simulink model "grid"  (R2023b)
settings: Solver=VariableStepAuto  StartTime=0.1  StopTime=180  RelTol=1e-3
values from neighbouring files (symbols this model uses):
  close_time = 40    [params.m]
  M1 = M1_backup    [automation.m]    (also in params.m = Machine)
  M2 = M1    [automation.m]    (also in params.m = Machine)
  open_time = 80    [params.m]
  Pn_L1 = M1.P0 + M2.P0    [params.m]
  Pn_L2 = Pn_L1 * 0.2    [params.m]
libraries: nesl_utility x21, ee_lib x21, fl_lib x10
settings Model: Creator=gosmann  LastModifiedBy=felipe

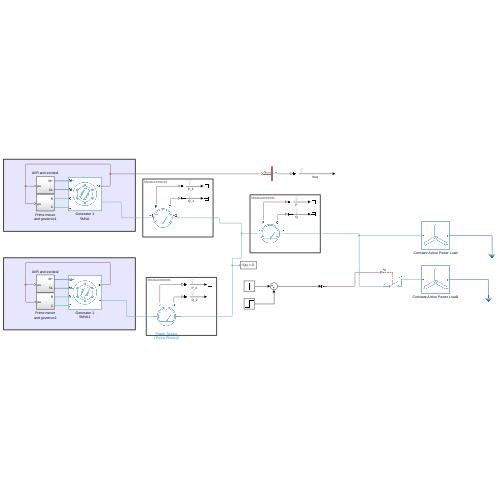
[thumbnail: Simulink's stored preview of the top-level diagram]
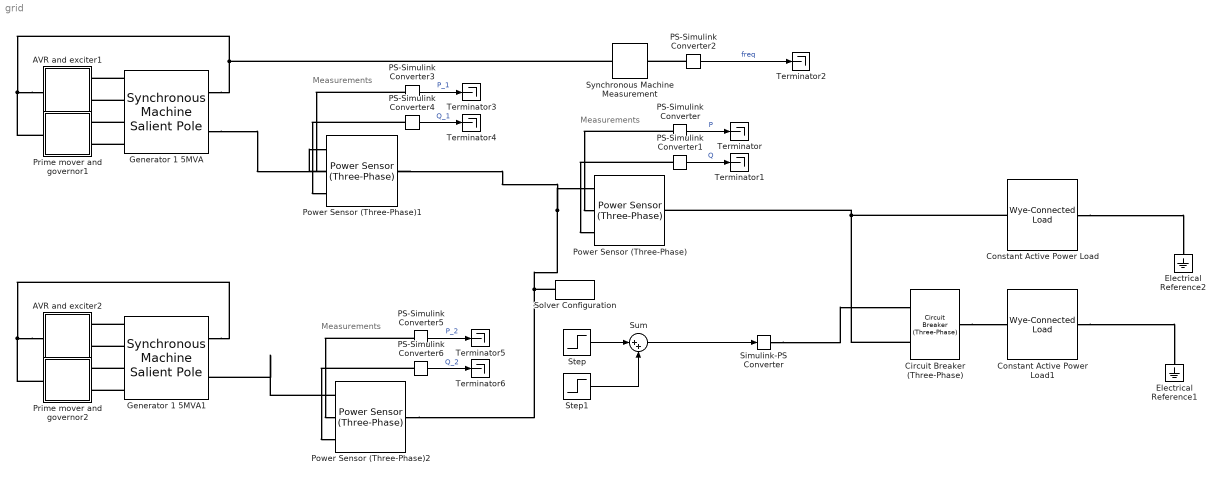
== system grid ==
  note: Measurements
  note: Measurements
  note: Measurements
  AVR and exciter1 : Subsystem
  AVR and exciter2 : Subsystem
  Circuit Breaker (Three-Phase) : ee_lib/Switches & Breakers/Circuit Breaker (Three-Phase)  R_closed=0.001 Ohm  G_open=1e-6 1/Ohm  threshold=0.5 V  breaker_behavior=ee.enum.switches.breakerBehavior.zeroCrossingEnable
      settings: InternalSimscapePortConfiguration="{\"Bottom\":[],\"Left\":[{\"id\":\"vT\",\"label\":\"vT\",\"type\":\"input\"},{\"id\":\"N1\",\"label\":\"~1\",\"type\":\"foundation.electrical.three_phase\"}],\"Right\":[{\"id\":\"N2\",\"label\":\"~2\",\"type\":\"foundation.electrical.three_phase\"}],\"Top\":[]}"
  Constant Active Power Load : ee_lib/Passive/RLC Assemblies/Wye-Connected Load  parameterization=ee.enum.rlc.parameterization.ratedpower  component_structure=ee.enum.rlc.structure.L  component_structure_PQ=ee.enum.rlc.structure.R  R=1 Ohm  L=7.3478 H  C=1e-6 F  VRated=ref_volt V  FRated=60 Hz  P=Pn_L1 W  Qpos=6000 A*V  Qneg=-1e2 A*V  R_parasitic=0 Ohm  G_parasitic=0 1/Ohm  R_parasitic_PQ=0 Ohm  G_parasitic_PQ=0 1/Ohm  Vmag0=4160*0.98 V  Vang0=0 deg  Freq0=60 Hz  IL_specify=off  IL_priority=High  IL=[0, 0, 0] A  IL_nominal_specify=off  IL_nominal_unit=A  IL_nominal_value=1  VC_specify=off  VC_priority=High  VC=[0, 0, 0] V  VC_nominal_specify=off  VC_nominal_unit=V  VC_nominal_value=1
  Constant Active Power Load1 : ee_lib/Passive/RLC Assemblies/Wye-Connected Load  parameterization=ee.enum.rlc.parameterization.ratedpower  component_structure=ee.enum.rlc.structure.L  component_structure_PQ=ee.enum.rlc.structure.R  R=1 Ohm  L=7.3478 H  C=1e-6 F  VRated=ref_volt V  FRated=60 Hz  P=Pn_L2 W  Qpos=6000 A*V  Qneg=-1e2 A*V  R_parasitic=0 Ohm  G_parasitic=0 1/Ohm  R_parasitic_PQ=0 Ohm  G_parasitic_PQ=0 1/Ohm  Vmag0=4160*0.98 V  Vang0=0 deg  Freq0=60 Hz  IL_specify=off  IL_priority=High  IL=[0, 0, 0] A  IL_nominal_specify=off  IL_nominal_unit=A  IL_nominal_value=1  VC_specify=off  VC_priority=High  VC=[0, 0, 0] V  VC_nominal_specify=off  VC_nominal_unit=V  VC_nominal_value=1
  Electrical Reference1 : fl_lib/Electrical/Electrical Elements/Electrical Reference
  Electrical Reference2 : fl_lib/Electrical/Electrical Elements/Electrical Reference
  Generator 1 5MVA : ee_lib/Electromechanical/Synchronous/Synchronous Machine Salient Pole  port_option=ee.enum.threePhasePort.composite  SRated=M1.Pn A*V  VRated=ref_volt V  FRated=ref_freq Hz  nPolePairs=M1.pole_pairs  param_option=ee.enum.sm.parameterization.standard  fieldCircuitParameterization_option=ee.enum.sm.fieldparameterization.current  baseEfd=216.54 V  baseIfd=M1.field_In A  zero_sequence=ee.enum.park.zerosequence.exclude  axes_param=ee.enum.rotorangle.daxis  Ladu=0.9  Laqu=0.55  L0=0.15  Ll=0.15  Ra=M1.Ra  Lfd=0.2571  Rfd=0.0006  L1d=0.2  R1d=0.0354  L1q=0.2567  R1q=0.0428  Xl=M1.Xi  Xd=M1.Xd  Xq=M1.Xq  X0=0.15  Xdd=M1.Xd_l  Xddd=M1.Xd_ll  Xqdd=M1.Xq_ll  d_option=ee.enum.circuit.open  Td0d=M1.Td0_l s  Tdd=1.75 s  Td0dd=M1.Td0_ll s  Tddd=0.0214 s  q_option=ee.enum.circuit.open  Tq0dd=M1.Tq0_ll s  Tqdd=0.0232 s  saturation_option=ee.enum.saturation.exclude  saturation_ifd=[0.00, 0.48, 0.76, 1.38, 1.79]  saturation_Vag=[0.00, 0.43, 0.59, 0.71, 0.76]  initialization_option=ee.enum.sm.initialization.electrical  source_type=ee.enum.sm.load_flow_source_type.Swing  Vmag0=ref_volt V  Vang0=0 deg  Pt0=M1.P0 A*V  Qt0=0 A*V  minimum_pu=0.95  phase_search_range=[-inf, inf] deg  gmin=1e-6 S  connection_option=ee.enum.Connection.wye  num_q_dampers=1  rotor_offset=-pi / 2 rad  pu_psid_specify=on  pu_psid_priority=High  pu_psid=0  pu_psid_nominal_specify=off  pu_psid_nominal_unit=1  pu_psid_nominal_value=1  pu_psiq_specify=on  pu_psiq_priority=High  pu_psiq=0  pu_psiq_nominal_specify=off  pu_psiq_nominal_unit=1  pu_psiq_nominal_value=1  pu_psifd_specify=on  pu_psifd_priority=High  pu_psifd=0  pu_psifd_nominal_specify=off  pu_psifd_nominal_unit=1  pu_psifd_nominal_value=1  pu_psi1d_specify=on  pu_psi1d_priority=High  pu_psi1d=0  pu_psi1d_nominal_specify=off  pu_psi1d_nominal_unit=1  pu_psi1d_nominal_value=1  pu_psi1q_specify=on  pu_psi1q_priority=High  pu_psi1q=0  pu_psi1q_nominal_specify=off  pu_psi1q_nominal_unit=1  pu_psi1q_nominal_value=1  angular_position_diff_specify=on  angular_position_diff_priority=High  angular_position_diff=0 deg  angular_position_diff_nominal_specify=off  angular_position_diff_nominal_unit=deg  angular_position_diff_nominal_value=1  Tmeas=298.15 K  alpha=3.93e-3 1/K  stator_thermal_mass=100 J/K  rotor_thermal_mass=200 J/K  temperatureA_specify=off  temperatureA_priority=High  temperatureA=25 degC  temperatureA_nominal_specify=off  temperatureA_nominal_unit=degC  temperatureA_nominal_value=1  temperatureB_specify=off  temperatureB_priority=High  temperatureB=25 degC  temperatureB_nominal_specify=off  temperatureB_nominal_unit=degC  temperatureB_nominal_value=1  temperatureC_specify=off  temperatureC_priority=High  temperatureC=25 degC  temperatureC_nominal_specify=off  temperatureC_nominal_unit=degC  temperatureC_nominal_value=1  temperatureR_specify=off  temperatureR_priority=High  temperatureR=25 degC  temperatureR_nominal_specify=off  temperatureR_nominal_unit=degC  temperatureR_nominal_value=1
      settings: LogSimulationData=on  InternalSimscapePortConfiguration="{\"Bottom\":[],\"Left\":[{\"id\":\"fd_p\",\"label\":\"fd+\",\"type\":\"foundation.electrical.electrical\"},{\"id\":\"fd_n\",\"label\":\"fd-\",\"type\":\"foundation.electrical.electrical\"},{\"id\":\"R\",\"label\":\"R\",\"type\":\"foundation.mechanical.rotational.rotational\"},{\"id\":\"C\",\"label\":\"C\",\"type\":\"foundation.mechanical.rotational.rotational\"}],\"Right\":[{\"id\":\"pu_output\",\"label\":\"pu\",\"type\":\"output\"},{\"id\":\"N\",\"label\":\"~\",\"type\":\"foundation.electrical.three_phase\"}],\"Top\":[]}"
  Generator 1 5MVA1 : ee_lib/Electromechanical/Synchronous/Synchronous Machine Salient Pole  port_option=ee.enum.threePhasePort.composite  SRated=M2.Pn A*V  VRated=ref_volt V  FRated=ref_freq Hz  nPolePairs=M2.pole_pairs  param_option=ee.enum.sm.parameterization.standard  fieldCircuitParameterization_option=ee.enum.sm.fieldparameterization.current  baseEfd=216.54 V  baseIfd=M2.field_In A  zero_sequence=ee.enum.park.zerosequence.exclude  axes_param=ee.enum.rotorangle.daxis  Ladu=0.9  Laqu=0.55  L0=0.15  Ll=0.15  Ra=M2.Ra  Lfd=0.2571  Rfd=0.0006  L1d=0.2  R1d=0.0354  L1q=0.2567  R1q=0.0428  Xl=M2.Xi  Xd=M2.Xd  Xq=M2.Xq  X0=0.15  Xdd=M2.Xd_l  Xddd=M2.Xd_ll  Xqdd=M2.Xq_ll  d_option=ee.enum.circuit.open  Td0d=M2.Td0_l s  Tdd=1.75 s  Td0dd=M2.Td0_ll s  Tddd=0.0214 s  q_option=ee.enum.circuit.open  Tq0dd=M2.Tq0_ll s  Tqdd=0.0232 s  saturation_option=ee.enum.saturation.exclude  saturation_ifd=[0.00, 0.48, 0.76, 1.38, 1.79]  saturation_Vag=[0.00, 0.43, 0.59, 0.71, 0.76]  initialization_option=ee.enum.sm.initialization.electrical  source_type=ee.enum.sm.load_flow_source_type.Swing  Vmag0=ref_volt V  Vang0=0 deg  Pt0=M2.P0 A*V  Qt0=0 A*V  minimum_pu=0.95  phase_search_range=[-inf, inf] deg  gmin=1e-6 S  connection_option=ee.enum.Connection.wye  num_q_dampers=1  rotor_offset=-pi / 2 rad  pu_psid_specify=on  pu_psid_priority=High  pu_psid=0  pu_psid_nominal_specify=off  pu_psid_nominal_unit=1  pu_psid_nominal_value=1  pu_psiq_specify=on  pu_psiq_priority=High  pu_psiq=0  pu_psiq_nominal_specify=off  pu_psiq_nominal_unit=1  pu_psiq_nominal_value=1  pu_psifd_specify=on  pu_psifd_priority=High  pu_psifd=0  pu_psifd_nominal_specify=off  pu_psifd_nominal_unit=1  pu_psifd_nominal_value=1  pu_psi1d_specify=on  pu_psi1d_priority=High  pu_psi1d=0  pu_psi1d_nominal_specify=off  pu_psi1d_nominal_unit=1  pu_psi1d_nominal_value=1  pu_psi1q_specify=on  pu_psi1q_priority=High  pu_psi1q=0  pu_psi1q_nominal_specify=off  pu_psi1q_nominal_unit=1  pu_psi1q_nominal_value=1  angular_position_diff_specify=on  angular_position_diff_priority=High  angular_position_diff=0 deg  angular_position_diff_nominal_specify=off  angular_position_diff_nominal_unit=deg  angular_position_diff_nominal_value=1  Tmeas=298.15 K  alpha=3.93e-3 1/K  stator_thermal_mass=100 J/K  rotor_thermal_mass=200 J/K  temperatureA_specify=off  temperatureA_priority=High  temperatureA=25 degC  temperatureA_nominal_specify=off  temperatureA_nominal_unit=degC  temperatureA_nominal_value=1  temperatureB_specify=off  temperatureB_priority=High  temperatureB=25 degC  temperatureB_nominal_specify=off  temperatureB_nominal_unit=degC  temperatureB_nominal_value=1  temperatureC_specify=off  temperatureC_priority=High  temperatureC=25 degC  temperatureC_nominal_specify=off  temperatureC_nominal_unit=degC  temperatureC_nominal_value=1  temperatureR_specify=off  temperatureR_priority=High  temperatureR=25 degC  temperatureR_nominal_specify=off  temperatureR_nominal_unit=degC  temperatureR_nominal_value=1
      settings: LogSimulationData=on  InternalSimscapePortConfiguration="{\"Bottom\":[],\"Left\":[{\"id\":\"fd_p\",\"label\":\"fd+\",\"type\":\"foundation.electrical.electrical\"},{\"id\":\"fd_n\",\"label\":\"fd-\",\"type\":\"foundation.electrical.electrical\"},{\"id\":\"R\",\"label\":\"R\",\"type\":\"foundation.mechanical.rotational.rotational\"},{\"id\":\"C\",\"label\":\"C\",\"type\":\"foundation.mechanical.rotational.rotational\"}],\"Right\":[{\"id\":\"pu_output\",\"label\":\"pu\",\"type\":\"output\"},{\"id\":\"N\",\"label\":\"~\",\"type\":\"foundation.electrical.three_phase\"}],\"Top\":[]}"
  PS-Simulink Converter{,1,3..6} (6 alike) : nesl_utility/PS-Simulink Converter  PhysicalDomain=network_engine_domain  SubClassName=ps_output  LeftPortType=input  RightPortType=output  PseudoPeriodic=off  Frequencies=[]  VectorFormat=1-D array  Unit=inherit  AffineConversion=off
  PS-Simulink Converter2 : nesl_utility/PS-Simulink Converter  PhysicalDomain=network_engine_domain  SubClassName=ps_output  LeftPortType=input  RightPortType=output  PseudoPeriodic=off  Frequencies=[]  VectorFormat=inherit  Unit=inherit  AffineConversion=off
  Power Sensor (Three-Phase) : ee_lib/Sensors & Transducers/Power Sensor (Three-Phase)  load_type=ee.enum.passive.type_balanced.balanced  f0=60 Hz  config=ee.enum.with_neutral.no  rho=1
      settings: InternalSimscapePortConfiguration="{\"Bottom\":[],\"Left\":[{\"id\":\"N1\",\"label\":\"~1\",\"type\":\"foundation.electrical.three_phase\"}],\"Right\":[{\"id\":\"N2\",\"label\":\"~2\",\"type\":\"foundation.electrical.three_phase\"}],\"Top\":[{\"id\":\"Pm\",\"label\":\"P\",\"type\":\"output\"},{\"id\":\"Qm\",\"label\":\"Q\",\"type\":\"output\"}]}"
  Power Sensor (Three-Phase)1 : ee_lib/Sensors & Transducers/Power Sensor (Three-Phase)  load_type=ee.enum.passive.type_balanced.balanced  f0=60 Hz  config=ee.enum.with_neutral.no  rho=1
      settings: InternalSimscapePortConfiguration="{\"Bottom\":[],\"Left\":[{\"id\":\"N1\",\"label\":\"~1\",\"type\":\"foundation.electrical.three_phase\"}],\"Right\":[{\"id\":\"N2\",\"label\":\"~2\",\"type\":\"foundation.electrical.three_phase\"}],\"Top\":[{\"id\":\"Pm\",\"label\":\"P\",\"type\":\"output\"},{\"id\":\"Qm\",\"label\":\"Q\",\"type\":\"output\"}]}"
  Power Sensor (Three-Phase)2 : ee_lib/Sensors & Transducers/Power Sensor (Three-Phase)  load_type=ee.enum.passive.type_balanced.balanced  f0=60 Hz  config=ee.enum.with_neutral.no  rho=1
      settings: InternalSimscapePortConfiguration="{\"Bottom\":[],\"Left\":[{\"id\":\"N1\",\"label\":\"~1\",\"type\":\"foundation.electrical.three_phase\"}],\"Right\":[{\"id\":\"N2\",\"label\":\"~2\",\"type\":\"foundation.electrical.three_phase\"}],\"Top\":[{\"id\":\"Pm\",\"label\":\"P\",\"type\":\"output\"},{\"id\":\"Qm\",\"label\":\"Q\",\"type\":\"output\"}]}"
  Prime mover and governor1 : Subsystem
  Prime mover and governor2 : Subsystem
  Simulink-PS Converter : nesl_utility/Simulink-PS Converter  PhysicalDomain=network_engine_domain  SubClassName=ps_input  LeftPortType=input  RightPortType=output  PseudoPeriodic=off  Frequencies=[]  NoiseDistribution=none  NoiseParameters=[]  Unit=1  AffineConversion=off  FilteringAndDerivatives=provide  SimscapeFilterOrder=1  InputFilterTimeConstant=0.001  UdotUserProvided=0
  Solver Configuration : nesl_utility/Solver Configuration  PhysicalDomain=network_engine_domain  SubClassName=solver  LeftPortType=input  RightPortType=generic  Tones=[]  Harmonics=[]  SimulateNoise=off  Profile=off  UseLocalSampling=off  EnableSwitchedLinearOptims=on  FrequencyDomain=off  UseCCode=off  RelTol=0.001  AbsTol=1e-06  MinStep=1e-09  ToWorkspace=off  RevertToSquareIcSolve=off  NumHomotopyIterations=100  PhasorMode=off  PhasorModeNumHarmonics=1  ConsistencySolver=NEWTON_FTOL  IndexReductionMethod=DerivativeReplacement  DoDC=off  ResidualTolerance=1e-09  ConsistencyTolSource=GLOBAL  ConsistencyAbsTol=0.001  ConsistencyRelTol=0.001  ConsistencyTolFactor=0.001  UseLocalSolver=on  LocalSolverChoice=NE_TRAPEZOIDAL_ADVANCER  ResolveIndetEquations=on  FunctionEvalNumThread=1  LocalSolverSampleTime=2e-4  DoFixedCost=on  MaxNonlinIter=1  MaxModeIter=2  ComputeImpulses=off  ImpulseIterations=1  LinearAlgebra=Full  LinearAlgebraNumThread=0  EquationFormulation=NE_TIME_EF  DelaysMemoryBudget=1024  AutomaticFiltering=on  FilteringTimeConstant=0.001  PartitionStorageMethod=AS_NEEDED  PartitionMemoryBudget=1024  PartitionMethod=ROBUST  MultibodyUseLocalSolver=off  MultibodyLocalSolverChoice=ODE1  MultibodyLocalSolverSampleTime=0.001
  Step : Step  Time=close_time  Before=1  After=0  SampleTime=0
  Step1 : Step  Time=open_time  SampleTime=0
  Sum : Sum  Inputs=|++
  Synchronous Machine Measurement : ee_lib/Electromechanical/Synchronous/Synchronous Machine Measurement  output_idx=4
      settings: InternalSimscapePortConfiguration="{\"Bottom\":[],\"Left\":[{\"id\":\"pu_input\",\"label\":\"pu\",\"type\":\"input\"}],\"Right\":[{\"id\":\"pu_output\",\"label\":\"o\",\"type\":\"output\"}],\"Top\":[]}"
  Terminator{,1..6} (7 alike) : Terminator
  wires:
  PS-Simulink Converter1/1 -> Terminator1/1  "Q"
  PS-Simulink Converter/1 -> Terminator/1  "P"
  PS-Simulink Converter2/1 -> Terminator2/1  "freq"
  Step/1 -> Sum/1
  Sum/1 -> Simulink-PS Converter/1
  Step1/1 -> Sum/2
  PS-Simulink Converter3/1 -> Terminator3/1  "P_1"
  PS-Simulink Converter4/1 -> Terminator4/1  "Q_1"
  PS-Simulink Converter5/1 -> Terminator5/1  "P_2"
  PS-Simulink Converter6/1 -> Terminator6/1  "Q_2"
  connections:
  Constant Active Power Load/LConn1 -- Circuit Breaker (Three-Phase)/LConn2 -- Power Sensor (Three-Phase)/RConn1
  Constant Active Power Load/RConn1 -- Electrical Reference2/LConn1
  PS-Simulink Converter/LConn1 -- Power Sensor (Three-Phase)/LConn2
  PS-Simulink Converter1/LConn1 -- Power Sensor (Three-Phase)/LConn3
  PS-Simulink Converter2/LConn1 -- Synchronous Machine Measurement/RConn1
  Constant Active Power Load1/RConn1 -- Electrical Reference1/LConn1
  Circuit Breaker (Three-Phase)/RConn1 -- Constant Active Power Load1/LConn1
  Simulink-PS Converter/RConn1 -- Circuit Breaker (Three-Phase)/LConn1
  AVR and exciter1/LConn1 -- Synchronous Machine Measurement/LConn1 -- Generator 1 5MVA/RConn1 -- Prime mover and governor1/LConn1
  Generator 1 5MVA/LConn1 -- AVR and exciter1/RConn1
  Generator 1 5MVA/LConn4 -- Prime mover and governor1/RConn2
  Generator 1 5MVA/LConn3 -- Prime mover and governor1/RConn1
  Generator 1 5MVA/LConn2 -- AVR and exciter1/RConn2
  AVR and exciter2/LConn1 -- Generator 1 5MVA1/RConn1 -- Prime mover and governor2/LConn1
  Generator 1 5MVA1/LConn1 -- AVR and exciter2/RConn1
  Generator 1 5MVA1/LConn3 -- Prime mover and governor2/RConn1
  Generator 1 5MVA1/LConn4 -- Prime mover and governor2/RConn2
  Generator 1 5MVA1/LConn2 -- AVR and exciter2/RConn2
  Solver Configuration/RConn1 -- Power Sensor (Three-Phase)1/RConn1 -- Power Sensor (Three-Phase)/LConn1 -- Power Sensor (Three-Phase)2/RConn1
  PS-Simulink Converter3/LConn1 -- Power Sensor (Three-Phase)1/LConn2
  PS-Simulink Converter4/LConn1 -- Power Sensor (Three-Phase)1/LConn3
  Generator 1 5MVA/RConn2 -- Power Sensor (Three-Phase)1/LConn1
  Power Sensor (Three-Phase)2/LConn1 -- Generator 1 5MVA1/RConn2
  PS-Simulink Converter5/LConn1 -- Power Sensor (Three-Phase)2/LConn2
  PS-Simulink Converter6/LConn1 -- Power Sensor (Three-Phase)2/LConn3

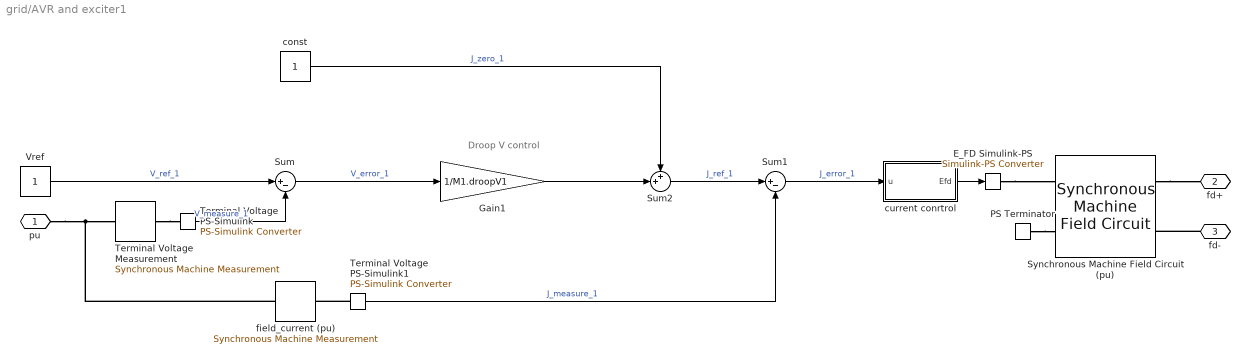
== system grid/AVR and exciter1 ==
  note: Droop V control
  "E_FD Simulink-PS " : nesl_utility/Simulink-PS Converter  PhysicalDomain=network_engine_domain  SubClassName=ps_input  LeftPortType=input  RightPortType=output  PseudoPeriodic=off  Frequencies=[]  NoiseDistribution=none  NoiseParameters=[]  Unit=1  AffineConversion=off  FilteringAndDerivatives=provide  SimscapeFilterOrder=1  InputFilterTimeConstant=.001  UdotUserProvided=0
  Gain1 : Gain  Gain=1/M1.droopV1
  PS Terminator : fl_lib/Physical Signals/Sinks/PS Terminator
  Sum : Sum  Inputs=|+-
  Sum1 : Sum  Inputs=|+-
  Sum2 : Sum  Inputs=++|
  Synchronous Machine Field Circuit (pu) : ee_lib/Electromechanical/Synchronous/Synchronous Machine Field Circuit  unit_option=ee.enum.unit.pu  SRated=M1.Pn V*A  FRated=ref_freq Hz  fieldCircuitParameterization_option=2  baseEfd=92.95 V  baseIfd=M1.field_In A  parameterization_option=2  Ladu=1.66  Rfd=0.0006  Xl=M1.Xi  Xd=M1.Xd  Xdd=M1.Xd_l  Xddd=M1.Xd_ll  d_option=ee.enum.circuit.open  Td0d=M1.Td0_l s  Tdd=1.3260 s  Td0dd=M1.Td0_ll s  Tddd=0.0230 s
      settings: LogSimulationData=on  InternalSimscapePortConfiguration="{\"Bottom\":[],\"Left\":[{\"id\":\"Efd_pu\",\"label\":\"Efd_pu\",\"type\":\"input\"},{\"id\":\"Ifd_pu\",\"label\":\"Ifd_pu\",\"type\":\"output\"}],\"Right\":[{\"id\":\"fd_p\",\"label\":\"fd+\",\"type\":\"foundation.electrical.electrical\"},{\"id\":\"fd_n\",\"label\":\"fd-\",\"type\":\"foundation.electrical.electrical\"}],\"Top\":[]}"
  Terminal Voltage Measurement : ee_lib/Electromechanical/Synchronous/Synchronous Machine Measurement  output_idx=14
      settings: LogSimulationData=on  InternalSimscapePortConfiguration="{\"Bottom\":[],\"Left\":[{\"id\":\"pu_input\",\"label\":\"pu\",\"type\":\"input\"}],\"Right\":[{\"id\":\"pu_output\",\"label\":\"o\",\"type\":\"output\"}],\"Top\":[]}"
  Terminal Voltage PS-Simulink : nesl_utility/PS-Simulink Converter  PhysicalDomain=network_engine_domain  SubClassName=ps_output  LeftPortType=input  RightPortType=output  PseudoPeriodic=off  Frequencies=[]  VectorFormat=1-D array  Unit=1  AffineConversion=off
  Terminal Voltage PS-Simulink1 : nesl_utility/PS-Simulink Converter  PhysicalDomain=network_engine_domain  SubClassName=ps_output  LeftPortType=input  RightPortType=output  PseudoPeriodic=off  Frequencies=[]  VectorFormat=1-D array  Unit=1  AffineConversion=off
  Vref : Constant
  const : Constant
  current conrtrol : Subsystem
  field_current (pu) : ee_lib/Electromechanical/Synchronous/Synchronous Machine Measurement  output_idx=2
      settings: InternalSimscapePortConfiguration="{\"Bottom\":[],\"Left\":[{\"id\":\"pu_input\",\"label\":\"pu\",\"type\":\"input\"}],\"Right\":[{\"id\":\"pu_output\",\"label\":\"o\",\"type\":\"output\"}],\"Top\":[]}"
  pu : PMIOPort  Side=Left
  fd+ : PMIOPort  Port=2  Side=Right
  fd- : PMIOPort  Port=3  Side=Right
  wires:
  Vref/1 -> Sum/1  "V_ref_1"
  current conrtrol/1(Efd) -> "E_FD Simulink-PS "/1
  Sum/1 -> Gain1/1  "V_error_1"
  const/1 -> Sum2/1  "J_zero_1"
  Sum1/1 -> current conrtrol/1(u)  "J_error_1"
  Terminal Voltage PS-Simulink1/1 -> Sum1/2  "J_measure_1"
  Terminal Voltage PS-Simulink/1 -> Sum/2  "V_measure_1"
  Sum2/1 -> Sum1/1  "J_ref_1"
  Gain1/1 -> Sum2/2
  connections:
  fd-/RConn1 -- Synchronous Machine Field Circuit (pu)/RConn2
  Synchronous Machine Field Circuit (pu)/RConn1 -- fd+/RConn1
  PS Terminator/LConn1 -- Synchronous Machine Field Circuit (pu)/LConn2
  "E_FD Simulink-PS "/RConn1 -- Synchronous Machine Field Circuit (pu)/LConn1
  field_current (pu)/LConn1 -- pu/RConn1 -- Terminal Voltage Measurement/LConn1
  Terminal Voltage Measurement/RConn1 -- Terminal Voltage PS-Simulink/LConn1
  Terminal Voltage PS-Simulink1/LConn1 -- field_current (pu)/RConn1

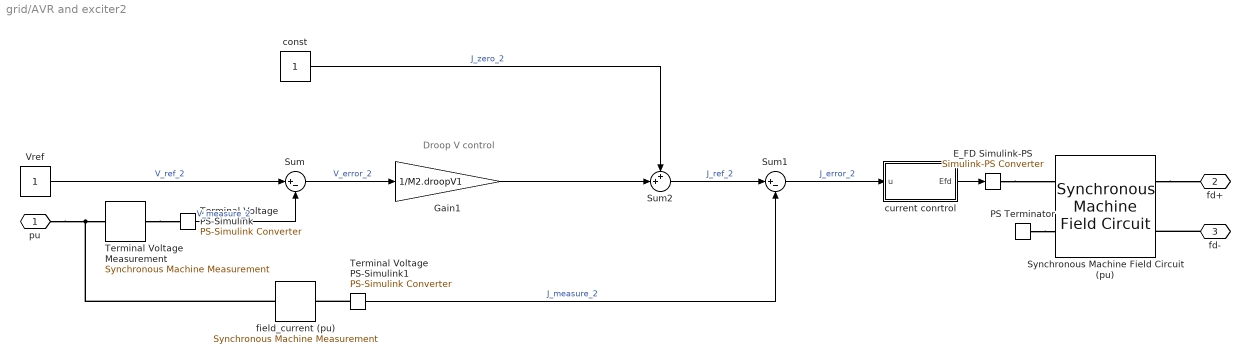
== system grid/AVR and exciter2 ==
  note: Droop V control
  "E_FD Simulink-PS " : nesl_utility/Simulink-PS Converter  PhysicalDomain=network_engine_domain  SubClassName=ps_input  LeftPortType=input  RightPortType=output  PseudoPeriodic=off  Frequencies=[]  NoiseDistribution=none  NoiseParameters=[]  Unit=1  AffineConversion=off  FilteringAndDerivatives=provide  SimscapeFilterOrder=1  InputFilterTimeConstant=.001  UdotUserProvided=0
  Gain1 : Gain  Gain=1/M2.droopV1
  PS Terminator : fl_lib/Physical Signals/Sinks/PS Terminator
  Sum : Sum  Inputs=|+-
  Sum1 : Sum  Inputs=|+-
  Sum2 : Sum  Inputs=++|
  Synchronous Machine Field Circuit (pu) : ee_lib/Electromechanical/Synchronous/Synchronous Machine Field Circuit  unit_option=ee.enum.unit.pu  SRated=M2.Pn V*A  FRated=ref_freq Hz  fieldCircuitParameterization_option=2  baseEfd=92.95 V  baseIfd=M2.field_In A  parameterization_option=2  Ladu=1.66  Rfd=0.0006  Xl=M2.Xi  Xd=M2.Xd  Xdd=M2.Xd_l  Xddd=M2.Xd_ll  d_option=ee.enum.circuit.open  Td0d=M2.Td0_l s  Tdd=1.3260 s  Td0dd=M2.Td0_ll s  Tddd=0.0230 s
      settings: LogSimulationData=on  InternalSimscapePortConfiguration="{\"Bottom\":[],\"Left\":[{\"id\":\"Efd_pu\",\"label\":\"Efd_pu\",\"type\":\"input\"},{\"id\":\"Ifd_pu\",\"label\":\"Ifd_pu\",\"type\":\"output\"}],\"Right\":[{\"id\":\"fd_p\",\"label\":\"fd+\",\"type\":\"foundation.electrical.electrical\"},{\"id\":\"fd_n\",\"label\":\"fd-\",\"type\":\"foundation.electrical.electrical\"}],\"Top\":[]}"
  Terminal Voltage Measurement : ee_lib/Electromechanical/Synchronous/Synchronous Machine Measurement  output_idx=14
      settings: LogSimulationData=on  InternalSimscapePortConfiguration="{\"Bottom\":[],\"Left\":[{\"id\":\"pu_input\",\"label\":\"pu\",\"type\":\"input\"}],\"Right\":[{\"id\":\"pu_output\",\"label\":\"o\",\"type\":\"output\"}],\"Top\":[]}"
  Terminal Voltage PS-Simulink : nesl_utility/PS-Simulink Converter  PhysicalDomain=network_engine_domain  SubClassName=ps_output  LeftPortType=input  RightPortType=output  PseudoPeriodic=off  Frequencies=[]  VectorFormat=1-D array  Unit=1  AffineConversion=off
  Terminal Voltage PS-Simulink1 : nesl_utility/PS-Simulink Converter  PhysicalDomain=network_engine_domain  SubClassName=ps_output  LeftPortType=input  RightPortType=output  PseudoPeriodic=off  Frequencies=[]  VectorFormat=1-D array  Unit=1  AffineConversion=off
  Vref : Constant
  const : Constant
  current conrtrol : Subsystem
  field_current (pu) : ee_lib/Electromechanical/Synchronous/Synchronous Machine Measurement  output_idx=2
      settings: InternalSimscapePortConfiguration="{\"Bottom\":[],\"Left\":[{\"id\":\"pu_input\",\"label\":\"pu\",\"type\":\"input\"}],\"Right\":[{\"id\":\"pu_output\",\"label\":\"o\",\"type\":\"output\"}],\"Top\":[]}"
  pu : PMIOPort  Side=Left
  fd+ : PMIOPort  Port=2  Side=Right
  fd- : PMIOPort  Port=3  Side=Right
  wires:
  Vref/1 -> Sum/1  "V_ref_2"
  current conrtrol/1(Efd) -> "E_FD Simulink-PS "/1
  Sum/1 -> Gain1/1  "V_error_2"
  const/1 -> Sum2/1  "J_zero_2"
  Sum1/1 -> current conrtrol/1(u)  "J_error_2"
  Terminal Voltage PS-Simulink1/1 -> Sum1/2  "J_measure_2"
  Terminal Voltage PS-Simulink/1 -> Sum/2  "V_measure_2"
  Sum2/1 -> Sum1/1  "J_ref_2"
  Gain1/1 -> Sum2/2
  connections:
  fd-/RConn1 -- Synchronous Machine Field Circuit (pu)/RConn2
  Synchronous Machine Field Circuit (pu)/RConn1 -- fd+/RConn1
  PS Terminator/LConn1 -- Synchronous Machine Field Circuit (pu)/LConn2
  "E_FD Simulink-PS "/RConn1 -- Synchronous Machine Field Circuit (pu)/LConn1
  field_current (pu)/LConn1 -- pu/RConn1 -- Terminal Voltage Measurement/LConn1
  Terminal Voltage Measurement/RConn1 -- Terminal Voltage PS-Simulink/LConn1
  Terminal Voltage PS-Simulink1/LConn1 -- field_current (pu)/RConn1

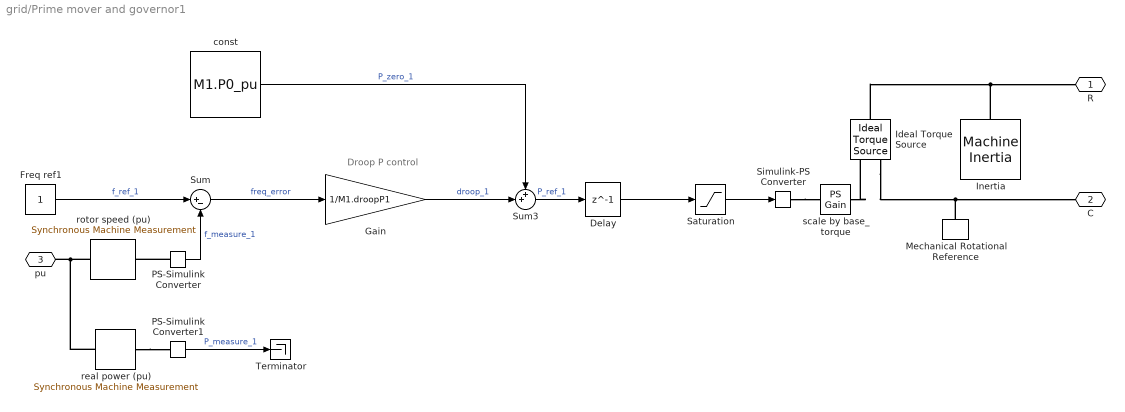
== system grid/Prime mover and governor1 ==
  note: Droop P control
  Delay : Delay  DelayLength=1
  Freq ref1 : Constant
  Gain : Gain  Gain=1/M1.droopP1
  Ideal Torque Source : fl_lib/Mechanical/Mechanical Sources/Ideal Torque Source
  Inertia : ee_lib/Electromechanical/Mechanical/Machine Inertia  SRated=M1.Pn V*A  FRated=ref_freq Hz  nPolePairs=M1.pole_pairs  inertia_option=1  J=M1.J kg*m^2  H=3.525 s*W/V/A  damper_option=2  D=39.0509 N*m/(rad/s)  pu_D=M1.damping  initialization_option=2  fMechanical0=60 Hz  fElectrical0=ref_freq Hz
      settings: LogSimulationData=on  InternalSimscapePortConfiguration="{\"Bottom\":[],\"Left\":[{\"id\":\"R\",\"label\":\"R\",\"type\":\"foundation.mechanical.rotational.rotational\"}],\"Right\":[],\"Top\":[]}"
  Mechanical Rotational Reference : fl_lib/Mechanical/Rotational Elements/Mechanical Rotational Reference
  PS-Simulink Converter : nesl_utility/PS-Simulink Converter  PhysicalDomain=network_engine_domain  SubClassName=ps_output  LeftPortType=input  RightPortType=output  PseudoPeriodic=off  Frequencies=[]  VectorFormat=1-D array  Unit=inherit  AffineConversion=off
  PS-Simulink Converter1 : nesl_utility/PS-Simulink Converter  PhysicalDomain=network_engine_domain  SubClassName=ps_output  LeftPortType=input  RightPortType=output  PseudoPeriodic=off  Frequencies=[]  VectorFormat=1-D array  Unit=inherit  AffineConversion=off
  Saturation : Saturate  UpperLimit=1  LowerLimit=0
  Simulink-PS Converter : nesl_utility/Simulink-PS Converter  PhysicalDomain=network_engine_domain  SubClassName=ps_input  LeftPortType=input  RightPortType=output  PseudoPeriodic=off  Frequencies=[]  NoiseDistribution=none  NoiseParameters=[]  Unit=1  AffineConversion=off  FilteringAndDerivatives=provide  SimscapeFilterOrder=1  InputFilterTimeConstant=0.001  UdotUserProvided=0
  Sum : Sum  Inputs=|+-
  Sum3 : Sum  Inputs=++|
  Terminator : Terminator
  const : Constant  Value=M1.P0_pu
  real power (pu) : ee_lib/Electromechanical/Synchronous/Synchronous Machine Measurement  output_idx=12
      settings: InternalSimscapePortConfiguration="{\"Bottom\":[],\"Left\":[{\"id\":\"pu_input\",\"label\":\"pu\",\"type\":\"input\"}],\"Right\":[{\"id\":\"pu_output\",\"label\":\"o\",\"type\":\"output\"}],\"Top\":[]}"
  rotor speed (pu) : ee_lib/Electromechanical/Synchronous/Synchronous Machine Measurement  output_idx=4
      settings: InternalSimscapePortConfiguration="{\"Bottom\":[],\"Left\":[{\"id\":\"pu_input\",\"label\":\"pu\",\"type\":\"input\"}],\"Right\":[{\"id\":\"pu_output\",\"label\":\"o\",\"type\":\"output\"}],\"Top\":[]}"
  scale by base_torque : fl_lib/Physical Signals/Functions/PS Gain  gain=M1.base_torque N*m
  R : PMIOPort  Side=Right
  C : PMIOPort  Port=2  Side=Right
  pu : PMIOPort  Port=3  Side=Left
  wires:
  PS-Simulink Converter/1 -> Sum/2  "f_measure_1"
  Freq ref1/1 -> Sum/1  "f_ref_1"
  Sum/1 -> Gain/1  "freq_error"
  PS-Simulink Converter1/1 -> Terminator/1  "P_measure_1"
  const/1 -> Sum3/1  "P_zero_1"
  Sum3/1 -> Delay/1  "P_ref_1"
  Saturation/1 -> Simulink-PS Converter/1
  Delay/1 -> Saturation/1
  Gain/1 -> Sum3/2  "droop_1"
  connections:
  scale by base_torque/RConn1 -- Ideal Torque Source/RConn1
  rotor speed (pu)/LConn1 -- real power (pu)/LConn1 -- pu/RConn1
  Ideal Torque Source/LConn1 -- Inertia/LConn1 -- R/RConn1
  Mechanical Rotational Reference/LConn1 -- Ideal Torque Source/RConn2 -- C/RConn1
  PS-Simulink Converter/LConn1 -- rotor speed (pu)/RConn1
  real power (pu)/RConn1 -- PS-Simulink Converter1/LConn1
  Simulink-PS Converter/RConn1 -- scale by base_torque/LConn1

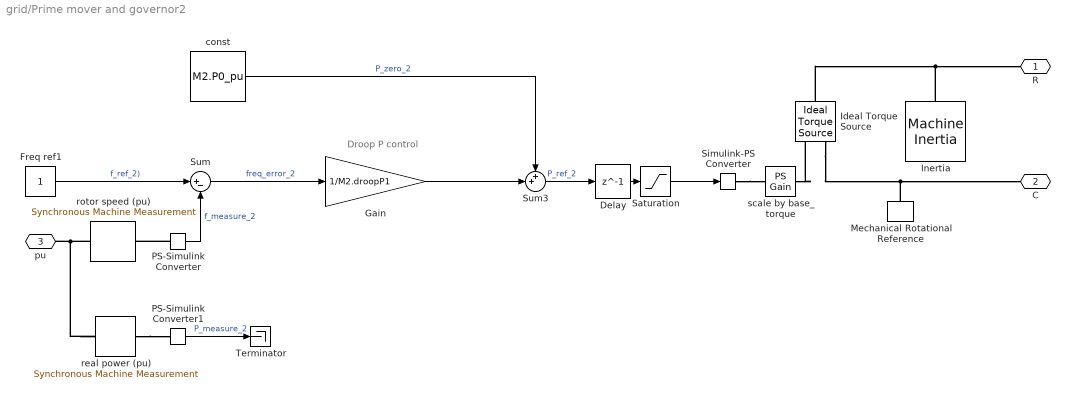
== system grid/Prime mover and governor2 ==
  note: Droop P control
  Delay : Delay  DelayLength=1
  Freq ref1 : Constant
  Gain : Gain  Gain=1/M2.droopP1
  Ideal Torque Source : fl_lib/Mechanical/Mechanical Sources/Ideal Torque Source
  Inertia : ee_lib/Electromechanical/Mechanical/Machine Inertia  SRated=M2.Pn V*A  FRated=ref_freq Hz  nPolePairs=M2.pole_pairs  inertia_option=1  J=M2.J kg*m^2  H=3.525 s*W/V/A  damper_option=2  D=39.0509 N*m/(rad/s)  pu_D=M2.damping  initialization_option=2  fMechanical0=60 Hz  fElectrical0=ref_freq Hz
      settings: LogSimulationData=on  InternalSimscapePortConfiguration="{\"Bottom\":[],\"Left\":[{\"id\":\"R\",\"label\":\"R\",\"type\":\"foundation.mechanical.rotational.rotational\"}],\"Right\":[],\"Top\":[]}"
  Mechanical Rotational Reference : fl_lib/Mechanical/Rotational Elements/Mechanical Rotational Reference
  PS-Simulink Converter : nesl_utility/PS-Simulink Converter  PhysicalDomain=network_engine_domain  SubClassName=ps_output  LeftPortType=input  RightPortType=output  PseudoPeriodic=off  Frequencies=[]  VectorFormat=1-D array  Unit=inherit  AffineConversion=off
  PS-Simulink Converter1 : nesl_utility/PS-Simulink Converter  PhysicalDomain=network_engine_domain  SubClassName=ps_output  LeftPortType=input  RightPortType=output  PseudoPeriodic=off  Frequencies=[]  VectorFormat=1-D array  Unit=inherit  AffineConversion=off
  Saturation : Saturate  UpperLimit=1  LowerLimit=0
  Simulink-PS Converter : nesl_utility/Simulink-PS Converter  PhysicalDomain=network_engine_domain  SubClassName=ps_input  LeftPortType=input  RightPortType=output  PseudoPeriodic=off  Frequencies=[]  NoiseDistribution=none  NoiseParameters=[]  Unit=1  AffineConversion=off  FilteringAndDerivatives=provide  SimscapeFilterOrder=1  InputFilterTimeConstant=0.001  UdotUserProvided=0
  Sum : Sum  Inputs=|+-
  Sum3 : Sum  Inputs=++|
  Terminator : Terminator
  const : Constant  Value=M2.P0_pu
  real power (pu) : ee_lib/Electromechanical/Synchronous/Synchronous Machine Measurement  output_idx=12
      settings: InternalSimscapePortConfiguration="{\"Bottom\":[],\"Left\":[{\"id\":\"pu_input\",\"label\":\"pu\",\"type\":\"input\"}],\"Right\":[{\"id\":\"pu_output\",\"label\":\"o\",\"type\":\"output\"}],\"Top\":[]}"
  rotor speed (pu) : ee_lib/Electromechanical/Synchronous/Synchronous Machine Measurement  output_idx=4
      settings: InternalSimscapePortConfiguration="{\"Bottom\":[],\"Left\":[{\"id\":\"pu_input\",\"label\":\"pu\",\"type\":\"input\"}],\"Right\":[{\"id\":\"pu_output\",\"label\":\"o\",\"type\":\"output\"}],\"Top\":[]}"
  scale by base_torque : fl_lib/Physical Signals/Functions/PS Gain  gain=M2.base_torque N*m
  R : PMIOPort  Side=Right
  C : PMIOPort  Port=2  Side=Right
  pu : PMIOPort  Port=3  Side=Left
  wires:
  PS-Simulink Converter/1 -> Sum/2  "f_measure_2"
  Freq ref1/1 -> Sum/1  "f_ref_2)"
  Sum/1 -> Gain/1  "freq_error_2"
  PS-Simulink Converter1/1 -> Terminator/1  "P_measure_2"
  const/1 -> Sum3/1  "P_zero_2"
  Sum3/1 -> Delay/1  "P_ref_2"
  Delay/1 -> Saturation/1
  Saturation/1 -> Simulink-PS Converter/1
  Gain/1 -> Sum3/2
  connections:
  scale by base_torque/RConn1 -- Ideal Torque Source/RConn1
  rotor speed (pu)/LConn1 -- real power (pu)/LConn1 -- pu/RConn1
  Ideal Torque Source/LConn1 -- Inertia/LConn1 -- R/RConn1
  Mechanical Rotational Reference/LConn1 -- Ideal Torque Source/RConn2 -- C/RConn1
  PS-Simulink Converter/LConn1 -- rotor speed (pu)/RConn1
  real power (pu)/RConn1 -- PS-Simulink Converter1/LConn1
  Simulink-PS Converter/RConn1 -- scale by base_torque/LConn1

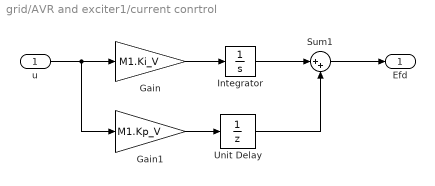
== system grid/AVR and exciter1/current conrtrol ==
  u : Inport
  Gain : Gain  Gain=M1.Ki_V
  Gain1 : Gain  Gain=M1.Kp_V
  Integrator : Integrator
  Sum1 : Sum  Inputs=|++
  Unit Delay : UnitDelay  InitialCondition=1  SampleTime=-1  HasFrameUpgradeWarning=on
  Efd : Outport
  wires:
  u/1 -> Gain1/1, Gain/1
  Sum1/1 -> Efd/1
  Gain/1 -> Integrator/1
  Integrator/1 -> Sum1/1
  Gain1/1 -> Unit Delay/1
  Unit Delay/1 -> Sum1/2

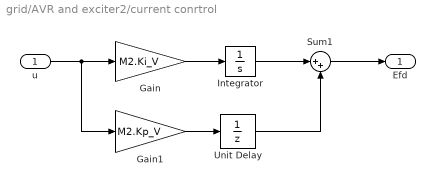
== system grid/AVR and exciter2/current conrtrol ==
  u : Inport
  Gain : Gain  Gain=M2.Ki_V
  Gain1 : Gain  Gain=M2.Kp_V
  Integrator : Integrator
  Sum1 : Sum  Inputs=|++
  Unit Delay : UnitDelay  InitialCondition=1  SampleTime=-1  HasFrameUpgradeWarning=on
  Efd : Outport
  wires:
  u/1 -> Gain1/1, Gain/1
  Sum1/1 -> Efd/1
  Gain/1 -> Integrator/1
  Integrator/1 -> Sum1/1
  Gain1/1 -> Unit Delay/1
  Unit Delay/1 -> Sum1/2
